simulink model "Full_Integration_Redundant"  (R2024b)
settings: Solver=VariableStepAuto  StartTime=0.0  StopTime=10.0  RelTol=1e-3
undefined symbols (not defined in the file): Bm1, Bm2, Br, Bsc, Btr, G, Im1, Im2, Isw, Jtr, Ke, Ke2, kp, kr, ks, Ksc, Kt, Kt2, ktr, Kv1, Kv2, L1, L2, lf, lr, Mr, N, n, n1, R1, R2, rp, Tfrc, to, Vx
libraries: simulink_extras x3, slpidlib x1
settings Model: Creator=Timothy  LastModifiedBy=HP
settings OptimizationCC: ReuseModelBlockBuffer=off
settings RTWCC: GPUComputeCapability=3.5

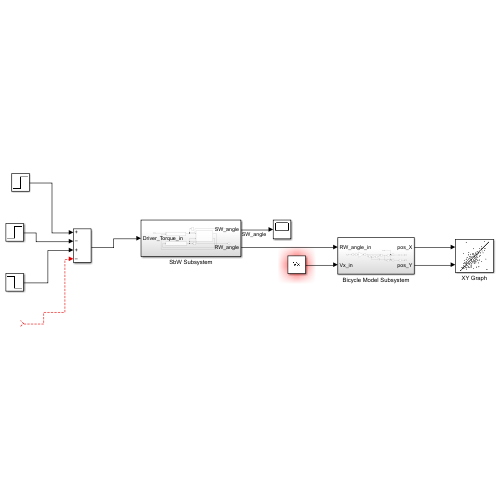
[thumbnail: Simulink's stored preview of the top-level diagram]
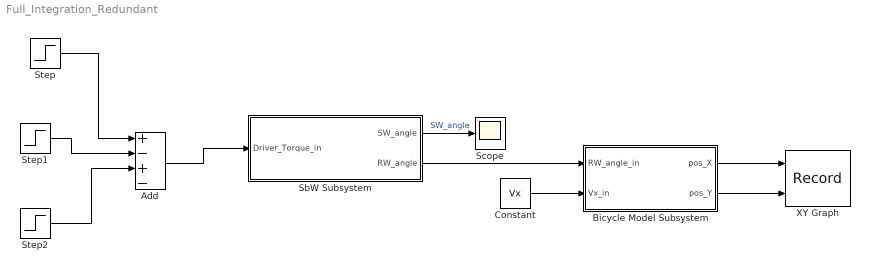
== system Full_Integration_Redundant ==
  Add : Sum  Inputs=+-+-
  Bicycle Model Subsystem : Subsystem
  Constant : Constant  Value=Vx
  SbW Subsystem : Subsystem
  Scope : Scope
  Step : Step  Time=30  After=0.5  SampleTime=0
  Step1 : Step  Time=30.1  After=0.5  SampleTime=0
  Step2 : Step  Time=60  After=-0.5  SampleTime=0
  XY Graph : Record  FileSettingsInternal="{\"entries\":[{\"content\":{\"excelSettings\":{\"content\":{},\"type\":\"Streamout.ExcelSettings\"}},\"type\":\"Streamout.FileSettingStorage\",\"uuid\":\"\"}],\"packageUris\":[\"http:\\/\\/schema.mathworks.com\\/mf0\\/streamout_blocks\\/R2020a\"],\"version\":\"1.0\"}"  Layout=[1 1]  SignalsInternal="{\"entries\":[{\"content\":{\"signals\":[{\"content\":{\"blockPath\":[],\"dimensions\":[1],\"domain\":\"\",\"lineColor\":\"#a2142f\",\"plots\":[ 1 ],\"port\":1,\"signalID\":1,\"signalName\":\"Bicycle Model Subsystem:1\"},\"type\":\"RecordBlkView.Signal\",\"uuid\":\"\"},{\"content\":{\"blockPath\":[],\"dimensions\":[1],\"domain\":\"\",\"lineColor\":\"#139fff\",\"plots\":[ 1 ],\"port\":2,\"signalID\":2,\"signalName\":\"Bicycle Model Subsystem:2\"},\"type\":\"RecordBlkView.Signal\",\"uuid\":\"\"}]},\"type\":\"RecordBlkView.InputSignals\",\"uuid\":\"\"}],\"packageUris\":[\"http:\\/\\/schema.mathworks.com\\/mf0\\/streamout_blocks\\/R2020a\"],\"version\":\"1.0\"}"  VisualizationBindings="{\"xyplotplugin\":{\"info\":[{\"series\":[{\"bindingParametersList\":[{\"parameter\":\"X-Axis\",\"signalID\":1,\"signalName\":\"Bicycle Model Subsystem:1\"},{\"parameter\":\"Y-Axis\",\"signalID\":2,\"signalName\":\"Bicycle Model Subsystem:2\"}],\"seriesID\":0}],\"subplotID\":1}]}}"  CompatibilityTag=XY
  wires:
  SbW Subsystem/1(SW_angle) -> Scope/1  "SW_angle"
  Add/1 -> SbW Subsystem/1(Driver_Torque_in)
  Bicycle Model Subsystem/1(pos_X) -> XY Graph/1
  SbW Subsystem/2(RW_angle) -> Bicycle Model Subsystem/1(RW_angle_in)
  Step/1 -> Add/1
  Step2/1 -> Add/3
  ? -> Add/4
  Constant/1 -> Bicycle Model Subsystem/2(Vx_in)
  Bicycle Model Subsystem/2(pos_Y) -> XY Graph/2
  Step1/1 -> Add/2

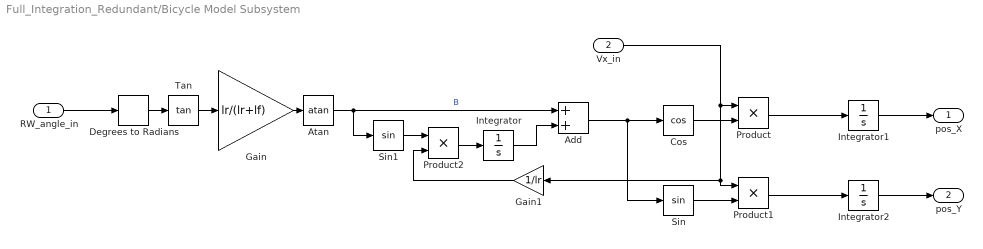
== system Full_Integration_Redundant/Bicycle Model Subsystem ==
  RW_angle_in : Inport
  Vx_in : Inport  Port=2
  Add : Sum
  Atan : Trigonometry  Operator=atan
  Cos : Trigonometry  Operator=cos
  Degrees to Radians : simulink_extras/Transformations/Degrees to Radians
  Gain : Gain  Gain=lr/(lr+lf)
  Gain1 : Gain  Gain=1/lr
  Integrator : Integrator
  Integrator1 : Integrator
  Integrator2 : Integrator
  Product : Product
  Product1 : Product
  Product2 : Product
  Sin : Trigonometry
  Sin1 : Trigonometry
  Tan : Trigonometry  Operator=tan
  pos_X : Outport
  pos_Y : Outport  Port=2
  wires:
  Degrees to Radians/1 -> Tan/1
  Product2/1 -> Integrator/1
  Cos/1 -> Product/2
  Add/1 -> Sin/1, Cos/1
  Atan/1 -> Add/1, Sin1/1  "B"
  Vx_in/1 -> Product1/1, Gain1/1, Product/1
  Integrator1/1 -> pos_X/1
  Gain1/1 -> Product2/2
  Integrator/1 -> Add/2
  Integrator2/1 -> pos_Y/1
  Gain/1 -> Atan/1
  Product/1 -> Integrator1/1
  Product1/1 -> Integrator2/1
  Tan/1 -> Gain/1
  RW_angle_in/1 -> Degrees to Radians/1
  Sin1/1 -> Product2/1
  Sin/1 -> Product1/2

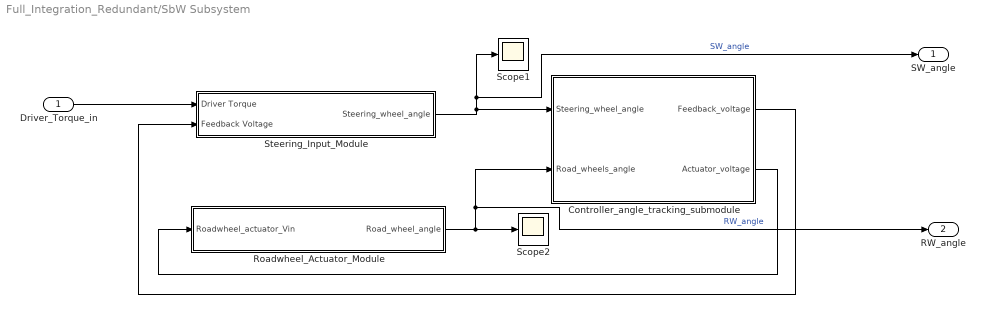
== system Full_Integration_Redundant/SbW Subsystem ==
  Driver_Torque_in : Inport
  Controller_angle_tracking_submodule : Subsystem
  Roadwheel_Actuator_Module : Subsystem
  Scope1 : Scope
  Scope2 : Scope
  Steering_Input_Module : Subsystem
  SW_angle : Outport
  RW_angle : Outport  Port=2
  wires:
  Roadwheel_Actuator_Module/1(Road_wheel_angle) -> Scope2/1, RW_angle/1, Controller_angle_tracking_submodule/2(Road_wheels_angle)  "RW_angle"
  Steering_Input_Module/1(Steering_wheel_angle) -> SW_angle/1, Scope1/1, Controller_angle_tracking_submodule/1(Steering_wheel_angle)  "SW_angle"
  Controller_angle_tracking_submodule/2(Actuator_voltage) -> Roadwheel_Actuator_Module/1(Roadwheel_actuator_Vin)
  Driver_Torque_in/1 -> Steering_Input_Module/1(Driver Torque)
  Controller_angle_tracking_submodule/1(Feedback_voltage) -> Steering_Input_Module/2(Feedback Voltage)

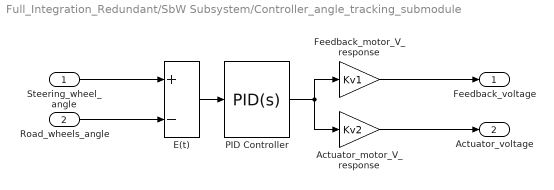
== system Full_Integration_Redundant/SbW Subsystem/Controller_angle_tracking_submodule ==
  Steering_wheel_angle : Inport
  Road_wheels_angle : Inport  Port=2
  Actuator_motor_V_response : Gain  Gain=Kv2
  E(t) : Sum  Inputs=+-
  Feedback_motor_V_response : Gain  Gain=Kv1
  PID Controller : slpidlib/PID Controller  Controller=PID  Form=Parallel  TimeDomain=Continuous-time  UseExternalTs=off  SampleTime=-1  IntegratorMethod=Forward Euler  FilterMethod=Forward Euler  ControllerParametersSource=internal  P=20  I=0.5  UseKiTs=off  D=-0.5  UseExternalDerivativeSource=off  N=100  UseFilter=on  TunerSelectOption=Transfer Function Based (PID Tuner App)  InitialConditionSource=internal  InitialConditionForIntegrator=0  InitialConditionForFilter=0  DifferentiatorICPrevScaledInput=0  ExternalReset=none  TrackingMode=off  Kt=1  LimitOutput=off  SatLimitsSource=internal  UpperSaturationLimit=100  LowerSaturationLimit=-100  LinearizeAsGain=on  AntiWindupMode=none  Kb=1  LimitIntegrator=off  UpperIntegratorSaturationLimit=inf  LowerIntegratorSaturationLimit=-inf  POutMin=[]  POutMax=[]  IOutMin=[]  IOutMax=[]  DOutMin=[]  DOutMax=[]  NOutMin=[]  NOutMax=[]  SumOutMin=[]  SumOutMax=[]  SaturationOutMin=[]  SaturationOutMax=[]  PParamMin=[]  PParamMax=[]  IParamMin=[]  IParamMax=[]  DParamMin=[]  DParamMax=[]  NParamMin=[]  NParamMax=[]  KbParamMin=[]  KbParamMax=[]  KtParamMin=[]  KtParamMax=[]  KbOutMin=[]  KbOutMax=[]  KtOutMin=[]  KtOutMax=[]  IntegratorOutMin=[]  IntegratorOutMax=[]  FilterOutMin=[]  FilterOutMax=[]  SumI1OutMin=[]  SumI1OutMax=[]  SumI2OutMin=[]  SumI2OutMax=[]  SumI3OutMin=[]  SumI3OutMax=[]  SumI4OutMin=[]  SumI4OutMax=[]  SumDOutMin=[]  SumDOutMax=[]  DifferentiatorOutMin=[]  DifferentiatorOutMax=[]  FilterDiffOutCoefMin=[]  FilterDiffOutCoefMax=[]  ReciprocalOutMin=[]  ReciprocalOutMax=[]  SumDenOutMin=[]  SumDenOutMax=[]  SumNumOutMin=[]  SumNumOutMax=[]  DivideOutMin=[]  DivideOutMax=[]  UdiffTsProdOutMin=[]  UdiffTsProdOutMax=[]  NTsProdOutMin=[]  NTsProdOutMax=[]  UintegralTsProdOutMin=[]  UintegralTsProdOutMax=[]  UngainTsProdOutMin=[]  UngainTsProdOutMax=[]  ClampingZeroOutDataTypeStr=Inherit: Inherit via back propagation  ClampingZeroOutMin=[]  ClampingZeroOutMax=[]  FilterDenConstantOutDataTypeStr=Inherit: Inherit via back propagation  FilterDenConstantOutMin=[]  FilterDenConstantOutMax=[]  PCopyOutDataTypeStr=Inherit: Inherit via back propagation  PCopyOutMin=[]  PCopyOutMax=[]  NCopyOutDataTypeStr=Inherit: Inherit via back propagation  NCopyOutMin=[]  NCopyOutMax=[]  IntegratorContinuousStateAttributes=''  IntegratorStateMustResolveToSignalObject=off  IntegratorRTWStateStorageClass=Auto  FilterContinuousStateAttributes=''  FilterStateMustResolveToSignalObject=off  FilterRTWStateStorageClass=Auto  ParallelPVariant=InternalParameters  IdealPVariant=Disabled  IVariant=InternalParameters  DVariant=InternalParameters  IntegratorVariant=Continuous  SatVariant=Disabled  AWVariant=Passthrough  PCopyVariant=Disabled  TRVariant=Disabled  FdbkBlocksVariant=Forward  IdealPFdbkVariant=Disabled  SatFdbkVariant=Disabled  DerivativeFilterVariant=ContFilter  NVariant=InternalParameters  NCopyVariant=Disabled  FilterICVariant=InternalICsFilter  IntegratorICVariant=InternalICs  ExternalResetVariant=Disabled  TRSumVariant=Passthrough  SumFdbkVariant=Disabled  SumVariant=Sum_PID  TsampFilterVariant=InternalTs  TsampNgainVariant=Passthrough  TsampIntegralVariant=Disabled_SignalSpec  ExternalSaturationOutDataTypeStr=Inherit: Same as second input  DerivativeSourceVariant=ErrorSignal  PreIntVariant=InternalPreInt
  Feedback_voltage : Outport
  Actuator_voltage : Outport  Port=2
  wires:
  Feedback_motor_V_response/1 -> Feedback_voltage/1
  E(t)/1 -> PID Controller/1
  PID Controller/1 -> Actuator_motor_V_response/1, Feedback_motor_V_response/1
  Road_wheels_angle/1 -> E(t)/2
  Steering_wheel_angle/1 -> E(t)/1
  Actuator_motor_V_response/1 -> Actuator_voltage/1

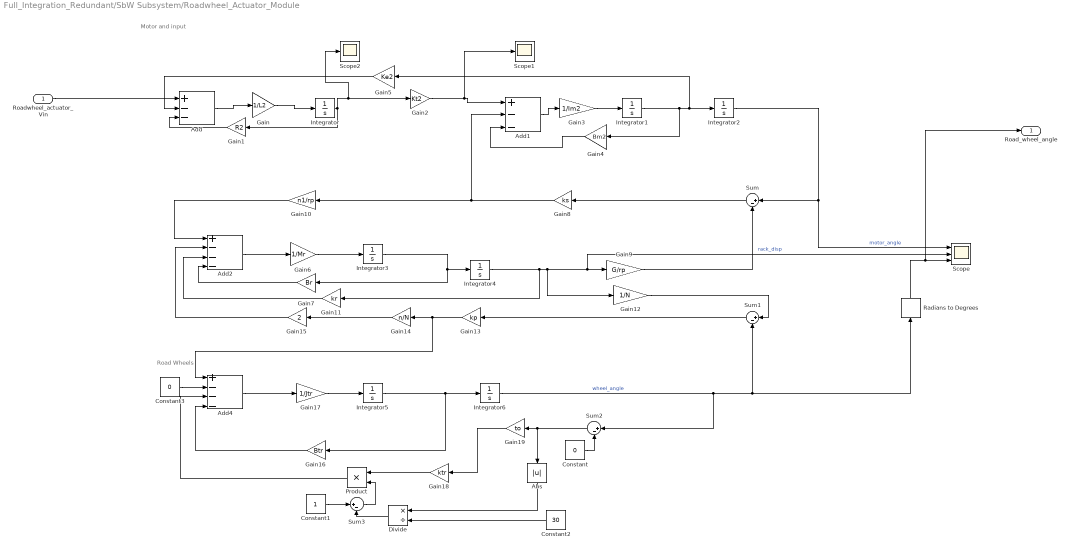
== system Full_Integration_Redundant/SbW Subsystem/Roadwheel_Actuator_Module ==
  note: Road Wheels
  note: Motor and input
  Roadwheel_actuator_Vin : Inport
  Abs : Abs  SaturateOnIntegerOverflow=off
  Add : Sum  Inputs=+--
  Add1 : Sum  Inputs=+--
  Add2 : Sum  Inputs=+---
  Add4 : Sum  Inputs=+---
  Constant : Constant  Value=0
  Constant1 : Constant
  Constant2 : Constant  Value=30
  Constant3 : Constant  Value=0
  Divide : Product  Inputs=*/
  Gain : Gain  Gain=1/L2
  Gain1 : Gain  Gain=R2
  Gain10 : Gain  Gain=n1/rp
  Gain11 : Gain  Gain=kr
  Gain12 : Gain  Gain=1/N
  Gain13 : Gain  Gain=kp
  Gain14 : Gain  Gain=n/N
  Gain15 : Gain  Gain=2
  Gain16 : Gain  Gain=Btr
  Gain17 : Gain  Gain=1/Jtr
  Gain18 : Gain  Gain=ktr
  Gain19 : Gain  Gain=to
  Gain2 : Gain  Gain=Kt2
  Gain3 : Gain  Gain=1/Im2
  Gain4 : Gain  Gain=Bm2
  Gain5 : Gain  Gain=Ke2
  Gain6 : Gain  Gain=1/Mr
  Gain7 : Gain  Gain=Br
  Gain8 : Gain  Gain=ks
  Gain9 : Gain  Gain=G/rp
  Integrator{,1..6} (7 alike) : Integrator
  Product : Product
  Radians to Degrees : simulink_extras/Transformations/Radians to Degrees
  Scope : Scope  NumInputPorts=3
  Scope1 : Scope
  Scope2 : Scope
  Sum{,1..3} (4 alike) : Sum  Inputs=|+-
  Road_wheel_angle : Outport
  wires:
  Gain11/1 -> Add2/3
  Abs/1 -> Divide/1
  Gain5/1 -> Add/2
  Integrator2/1 -> Sum/1, Scope/1  "motor_angle"
  Add1/1 -> Gain3/1
  Gain2/1 -> Scope1/1, Add1/1
  Gain3/1 -> Integrator1/1
  Gain13/1 -> Add4/1, Gain14/1
  Integrator6/1 -> Radians to Degrees/1, Sum1/2, Sum2/1  "wheel_angle"
  Gain6/1 -> Integrator3/1
  Constant1/1 -> Sum3/1
  Roadwheel_actuator_Vin/1 -> Add/1
  Divide/1 -> Sum3/2
  Gain10/1 -> Add2/1
  Integrator/1 -> Gain1/1, Gain2/1, Scope2/1
  Gain1/1 -> Add/3
  Add4/1 -> Gain17/1
  Add/1 -> Gain/1
  Integrator1/1 -> Gain4/1, Gain5/1, Integrator2/1
  Constant2/1 -> Divide/2
  Sum/1 -> Gain8/1
  Sum3/1 -> Product/2
  Gain12/1 -> Sum1/1
  Gain19/1 -> Gain18/1
  Gain15/1 -> Add2/2
  Product/1 -> Add4/3
  Gain18/1 -> Product/1
  Integrator4/1 -> Gain11/1, Gain12/1, Scope/2, Gain9/1  "rack_disp"
  Sum2/1 -> Abs/1, Gain19/1
  Gain9/1 -> Sum/2
  Add2/1 -> Gain6/1
  Integrator3/1 -> Gain7/1, Integrator4/1
  Constant3/1 -> Add4/2
  Gain4/1 -> Add1/3
  Integrator5/1 -> Gain16/1, Integrator6/1
  Gain14/1 -> Gain15/1
  Constant/1 -> Sum2/2
  Sum1/1 -> Gain13/1
  Radians to Degrees/1 -> Road_wheel_angle/1, Scope/3
  Gain16/1 -> Add4/4
  Gain8/1 -> Gain10/1, Add1/2
  Gain17/1 -> Integrator5/1
  Gain/1 -> Integrator/1
  Gain7/1 -> Add2/4

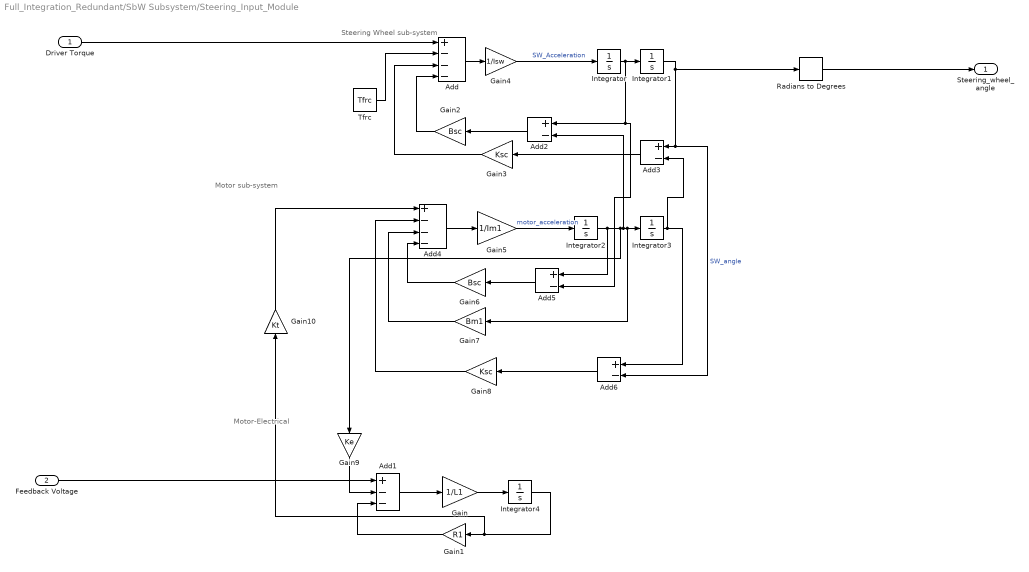
== system Full_Integration_Redundant/SbW Subsystem/Steering_Input_Module ==
  note: Steering Wheel sub-system
  note: Motor-Electrical
  note: Motor sub-system
  Driver Torque : Inport
  Feedback Voltage : Inport  Port=2
  Add : Sum  Inputs=+---
  Add1 : Sum  Inputs=+--
  Add{2..3,5..6} (4 alike) : Sum  Inputs=+-
  Add4 : Sum  Inputs=+---
  Gain : Gain  Gain=1/L1
  Gain1 : Gain  Gain=R1
  Gain10 : Gain  Gain=Kt
  Gain2 : Gain  Gain=Bsc
  Gain3 : Gain  Gain=Ksc
  Gain4 : Gain  Gain=1/Isw
  Gain5 : Gain  Gain=1/Im1
  Gain6 : Gain  Gain=Bsc
  Gain7 : Gain  Gain=Bm1
  Gain8 : Gain  Gain=Ksc
  Gain9 : Gain  Gain=Ke
  Integrator{,1..4} (5 alike) : Integrator
  Radians to Degrees : simulink_extras/Transformations/Radians to Degrees
  Tfrc : Constant  Value=Tfrc
  Steering_wheel_angle : Outport
  wires:
  Gain2/1 -> Add/4
  Integrator1/1 -> Add6/2, Add3/1, Radians to Degrees/1  "SW_angle"
  Gain10/1 -> Add4/1
  Gain6/1 -> Add4/4
  Gain8/1 -> Add4/2
  Tfrc/1 -> Add/2
  Gain1/1 -> Add1/3
  Integrator/1 -> Integrator1/1, Add2/1, Add5/2
  Add3/1 -> Gain3/1
  Integrator3/1 -> Add3/2, Add6/1
  Integrator2/1 -> Gain9/1, Add2/2, Gain7/1, Integrator3/1, Add5/1
  Add/1 -> Gain4/1
  Add6/1 -> Gain8/1
  Feedback Voltage/1 -> Add1/1
  Gain/1 -> Integrator4/1
  Gain5/1 -> Integrator2/1  "motor_acceleration"
  Gain7/1 -> Add4/3
  Add1/1 -> Gain/1
  Gain3/1 -> Add/3
  Integrator4/1 -> Gain1/1, Gain10/1
  Add2/1 -> Gain2/1
  Add4/1 -> Gain5/1
  Driver Torque/1 -> Add/1
  Add5/1 -> Gain6/1
  Radians to Degrees/1 -> Steering_wheel_angle/1
  Gain9/1 -> Add1/2
  Gain4/1 -> Integrator/1  "SW_Acceleration"
